simulink model "trim"  (R2015b)
settings: Solver=VariableStepAuto  StartTime=0.0  StopTime=4  RelTol=1e-3
undefined symbols (not defined in the file): alpharad, C_D_0, C_L_0, C_L_alpha, C_L_delta_e, C_M_0, C_M_alpha, C_M_delta_e, g, k, m, rho, S_ref, V, w
settings Model: Creator=Pramod  LastModifiedBy=Pramod

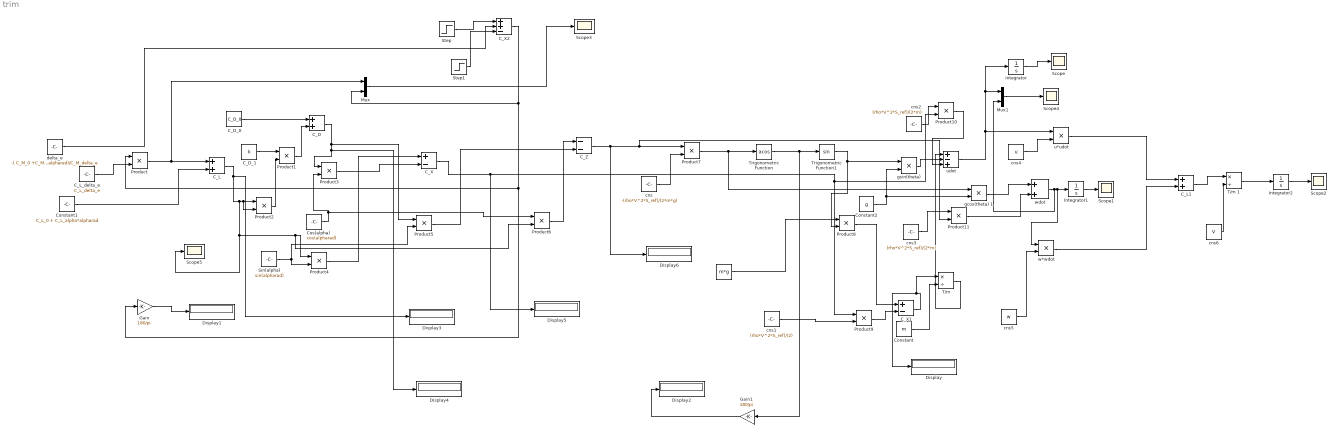
== system trim ==
  " " : Constant  Value=m*g
  C_D : Sum
  C_D_0 : Constant  Value=C_D_0
  C_D_1 : Constant  Value=k
  C_L : Sum
  C_L1 : Sum
  C_L_delta_e : Constant  Value=C_L_delta_e
  C_X : Sum  Inputs=+-
  C_X1 : Sum  Inputs=+-
  C_X2 : Sum  Inputs=++-
  C_Z : Sum  Inputs=--
  Constant : Constant  Value=m
  Constant1 : Constant  Value=C_L_0 + C_L_alpha*alpharad
  Constant2 : Constant  Value=g
  Cos(alpha) : Constant  Value=cos(alpharad)
  Display{,1..6} (7 alike) : Display
  Gain : Gain  Gain=180/pi
  Gain1 : Gain  Gain=180/pi
  Integrator : Integrator  InitialCondition=u
  Integrator1 : Integrator  InitialCondition=w
  Integrator2 : Integrator  InitialCondition=V
  Mux : Mux  Inputs=2
  Mux1 : Mux  Inputs=2
  Product{,1..11} (12 alike) : Product
  Scope{,1..5} (6 alike) : Scope
  Sin(alpha) : Constant  Value=sin(alpharad)
  Step : Step  Time=3  After=-5*pi/180  SampleTime=0
  Step1 : Step  Time=3.5  After=-5*pi/180  SampleTime=0
  "T/m " : Product  Inputs=*/
  T/m 1 : Product  Inputs=*/
  Trigonometric Function : Trigonometry  Operator=acos
  Trigonometric Function1 : Trigonometry
  cns : Constant  Value=-(rho*V^2*S_ref)/(2*m*g)
  cns1 : Constant  Value=(rho*V^2*S_ref)/(2)
  cns2 : Constant  Value=(rho*V^2*S_ref)/(2*m)
  cns3 : Constant  Value=(rho*V^2*S_ref)/(2*m)
  cns4 : Constant  Value=u
  cns5 : Constant  Value=w
  cns6 : Constant  Value=V
  delta_e : Constant  Value=-( C_M_0 +C_M_alpha*alpharad)/C_M_delta_e
  gcos(theta) 1 : Product
  "gsin(theta) " : Product
  u*udot : Product
  "udot " : Sum  Inputs=+-+
  w*wdot : Product
  wdot : Sum
  wires:
  C_L_delta_e/1 -> Product/2
  Product/1 -> Mux/1, C_L/1
  Constant1/1 -> C_L/2
  C_D_1/1 -> Product1/1
  C_L/1 -> Display3/1, Scope5/1, Product6/2, Product4/1, Product2/2, Product2/1
  Product2/1 -> Product1/2
  C_D_0/1 -> C_D/1
  Product1/1 -> C_D/2
  C_D/1 -> Display4/1, Product3/1, Product5/1
  Cos(alpha)/1 -> Product6/1, Product3/2
  Sin(alpha)/1 -> Product5/2, Product4/2
  Product3/1 -> C_X/2
  Product4/1 -> C_X/1
  Product6/1 -> C_Z/1
  Product5/1 -> C_Z/2
  cns/1 -> Product7/2
  C_Z/1 -> Display6/1, Product11/2, Product7/1
  Product7/1 -> gcos(theta) 1/1, Trigonometric Function/1
  Trigonometric Function/1 -> Gain1/1, Trigonometric Function1/1
  " "/1 -> Product8/1
  Trigonometric Function1/1 -> "gsin(theta) "/1, Product8/2
  cns1/1 -> Product9/2
  C_X/1 -> Display5/1, Product10/2, Product9/1
  Product9/1 -> C_X1/2
  Product8/1 -> C_X1/1
  C_X1/1 -> "T/m "/1, Display/1
  Gain/1 -> Display1/1
  Gain1/1 -> Display2/1
  Constant/1 -> "T/m "/2
  Constant2/1 -> gcos(theta) 1/2, "gsin(theta) "/2
  cns2/1 -> Product10/1
  "T/m "/1 -> "udot "/1
  "gsin(theta) "/1 -> "udot "/2
  Product10/1 -> "udot "/3
  cns3/1 -> Product11/1
  gcos(theta) 1/1 -> wdot/1
  Product11/1 -> wdot/2
  "udot "/1 -> u*udot/1, Mux1/1, Integrator/1
  wdot/1 -> Mux1/2, w*wdot/1, Integrator1/1
  Integrator/1 -> Scope/1
  Integrator1/1 -> Scope1/1
  cns4/1 -> u*udot/2
  cns5/1 -> w*wdot/2
  u*udot/1 -> C_L1/1
  w*wdot/1 -> C_L1/2
  C_L1/1 -> T/m 1/1
  cns6/1 -> T/m 1/2
  T/m 1/1 -> Integrator2/1
  Integrator2/1 -> Scope2/1
  Step/1 -> C_X2/1
  Step1/1 -> C_X2/3
  delta_e/1 -> C_X2/2
  C_X2/1 -> Gain/1, Product/1, Mux/2
  Mux/1 -> Scope3/1
  Mux1/1 -> Scope4/1
